simulink model "Modelo_R2023b"  (R2023b)
settings: Solver=VariableStepAuto  StartTime=0.0  StopTime=10.0  RelTol=1e-3
model workspace (MAT data in the model file):
  DC_Joint_J = 0.192319441127
  DC_Motor_D = 0.4
  DC_Motor_H = 0.192915716702
  DC_Motor_I = 1
  DC_Motor_J = 0.2131632295
  DC_Motor_Lower_Sat_Ref = -18
  DC_Motor_NLC = 0.11
  DC_Motor_NLS = 10000
  DC_Motor_P = 0.20625
  DC_Motor_ST = 0.0494309
  DC_Motor_TG = 0.95
  DC_Motor_Upper_Sat_Ref = 18
  DC_Motor_V = 12
  DRV_Deadzone_U = 128
  DRV_Motor_BTH = 0.001
  DRV_Motor_ETH = 0.15625
  DRV_Motor_FDR = 0.195188957589
  DRV_Motor_RTH = 0.001
  DRV_Motor_TBR = 0.10371374274
  MOTOR_Period_T = 0.01
  MOTOR_WHEEL_LPF : object (value not decoded)
  Robot_L = 0.15
  Robot_W = 0.15
  Robot_init_th = 0
  Robot_init_x = 0
  Robot_init_y = 0
  Robot_mm_to_m = 0.001
  Robot_wheel_radius = 0.05
  Robot_wheel_x_offset = 150
  Robot_wheel_y_offset = 102.5
  Robot_wheel_z_offset = 2
  Roller_Contact_df = 0.3
  Roller_Contact_dm = 1000
  Roller_Contact_sf = 0.5
  Roller_Contact_st = 1000000
  Roller_Joint_Friction = 0
  SIM_Base_Period_T = 0.001
  SIM_CTRL_Period_T = 0.1
  SIM_Floor_Height = 8.7
  SIM_Floor_Thick = 0.2
  SIM_Floor_Width = 9
  Sig : Simulink.Signal (value not decoded)
  Traj_ref = [0 0.1 0.2 0.3 0.4 0.5 0.6 0.7 0.8 0.9 1 0 ... (22 elements, 11x2)]
undefined symbols (not defined in the file): DiscIntNeverNeededParam, X, Y, Z
libraries: sm_lib x185, nesl_utility x37, fl_lib x32, ee_lib x12, simulink x8, aerolibconvert2 x4, cstblocks x4, sharedtransform x1, dspsigops x1
(part 2 of 4)

== system Modelo_R2023b/Nexus/World Frame with gravity ==
  Mechanism Configuration : sm_lib/Utilities/Mechanism Configuration  UniformGravity=Constant  GravityVector=[0 0 -9.80665]  GravityVectorUnits=m/s^2  LinearizationDelta=0.001  JointModeTransitionNonlinearIterations=2
  Solver Configuration : nesl_utility/Solver Configuration  PhysicalDomain=network_engine_domain  SubClassName=solver  LeftPortType=input  RightPortType=generic  Tones=[]  Harmonics=[]  SimulateNoise=off  Profile=off  UseLocalSampling=off  EnableSwitchedLinearOptims=on  FrequencyDomain=off  UseCCode=off  RelTol=0.001  AbsTol=1e-06  MinStep=1e-09  ToWorkspace=off  RevertToSquareIcSolve=off  NumHomotopyIterations=100  PhasorMode=off  PhasorModeNumHarmonics=1  ConsistencySolver=NEWTON_FTOL  IndexReductionMethod=DerivativeReplacement  DoDC=on  ResidualTolerance=1e-09  ConsistencyTolSource=GLOBAL  ConsistencyAbsTol=0.001  ConsistencyRelTol=0.001  ConsistencyTolFactor=0.001  UseLocalSolver=on  LocalSolverChoice=NE_PARTITIONING_ADVANCER  ResolveIndetEquations=on  FunctionEvalNumThread=1  LocalSolverSampleTime=0.001  DoFixedCost=off  MaxNonlinIter=3  MaxModeIter=2  ComputeImpulses=off  ImpulseIterations=2  LinearAlgebra=auto  LinearAlgebraNumThread=0  EquationFormulation=NE_TIME_EF  DelaysMemoryBudget=1024  AutomaticFiltering=off  FilteringTimeConstant=0.001  PartitionStorageMethod=AS_NEEDED  PartitionMemoryBudget=1024  PartitionMethod=FAST  MultibodyUseLocalSolver=off  MultibodyLocalSolverChoice=ODE1  MultibodyLocalSolverSampleTime=0.001
  World Frame : sm_lib/Frames and Transforms/World Frame
  WF : PMIOPort  Side=Right
  connections:
  Mechanism Configuration/RConn1 -- WF/RConn1 -- World Frame/RConn1 -- Solver Configuration/RConn1

== system Modelo_R2023b/Nexus/Nexus Robot/Sensors ==
  Frontal_Sonar_Sensor : sm_lib/Body Elements/File Solid  ExtGeomFileName=c_Nexus_Sonar_Sensor.stl  UnitType=Custom  ExtGeomFileUnits=mm  StepReaderType=HEX  ExportConvexHullGeometry=off  InertiaType=Custom  Mass=0  MassUnits=kg  CenterOfMass=[0, 0, 0]  CenterOfMassUnits=m  MomentsOfInertia=[0, 0, 0]  MomentsOfInertiaUnits=kg*m^2  ProductsOfInertia=[0, 0, 0]  ProductsOfInertiaUnits=kg*m^2  BasedOnType=DensityFromFile  Density=1000  DensityUnits=kg/m^3  DoExposeReferenceFrame=on  SerializedFrames=<Frames/>  GraphicType=FromGeometry  MarkerShape=Sphere  MarkerSize=10  GraphicVisPropType=SimpleVisualProperties  GraphicDiffuseColor=[0.15, 0.15, 0.15]  GraphicSpecularColor=[0.5 0.5 0.5 1.0]  GraphicAmbientColor=[0.15 0.15 0.15 1.0]  GraphicEmissiveColor=[0.0 0.0 0.0 1.0]  GraphicShininess=75  GraphicOpacity=1
  Left_Sonar_Sensor : sm_lib/Body Elements/File Solid  ExtGeomFileName=c_Nexus_Sonar_Sensor.stl  UnitType=Custom  ExtGeomFileUnits=mm  StepReaderType=HEX  ExportConvexHullGeometry=off  InertiaType=Custom  Mass=0  MassUnits=kg  CenterOfMass=[0, 0, 0]  CenterOfMassUnits=m  MomentsOfInertia=[0, 0, 0]  MomentsOfInertiaUnits=kg*m^2  ProductsOfInertia=[0, 0, 0]  ProductsOfInertiaUnits=kg*m^2  BasedOnType=DensityFromFile  Density=1000  DensityUnits=kg/m^3  DoExposeReferenceFrame=on  SerializedFrames=<Frames/>  GraphicType=FromGeometry  MarkerShape=Sphere  MarkerSize=10  GraphicVisPropType=SimpleVisualProperties  GraphicDiffuseColor=[0.15, 0.15, 0.15]  GraphicSpecularColor=[0.5 0.5 0.5 1.0]  GraphicAmbientColor=[0.15 0.15 0.15 1.0]  GraphicEmissiveColor=[0.0 0.0 0.0 1.0]  GraphicShininess=75  GraphicOpacity=1
  RT_Sensor_derecho : sm_lib/Frames and Transforms/Rigid Transform  TranslationMethod=Cartesian  TranslationStandardOffset=0  TranslationStandardOffsetUnits=m  TranslationStandardAxis=+Z  TranslationCartesianOffset=[0, -0.108, 0.01]  TranslationCartesianOffsetUnits=m  TranslationROffset=0  TranslationROffsetUnits=m  TranslationZOffset=0  TranslationZOffsetUnits=m  TranslationThetaOffset=0  TranslationThetaOffsetUnits=deg  RotationMethod=RotationSequence  RotationAngleUnits=deg  RotationStandardAxis=+Z  RotationAngle=0.0  RotationArbitraryAxis=[0 0 1]  FollAlignAxisA=+X  BaseAlignAxisA=+Y  FollAlignAxisB=+Y  BaseAlignAxisB=+Z  RotationSequenceAxes=BaseAxes  RotationSequence=ZYX  RotationSequenceAngles=[-90, 90, 0]  RotationSequenceAnglesUnits=deg  RotationMatrix=[1 0 0; 0 1 0; 0 0 1]  Quaternion=[1 0 0 0]
  RT_Sensor_frontal : sm_lib/Frames and Transforms/Rigid Transform  TranslationMethod=Cartesian  TranslationStandardOffset=0  TranslationStandardOffsetUnits=m  TranslationStandardAxis=+Z  TranslationCartesianOffset=[0.205, 0, 0.01]  TranslationCartesianOffsetUnits=m  TranslationROffset=0  TranslationROffsetUnits=m  TranslationZOffset=0  TranslationZOffsetUnits=m  TranslationThetaOffset=0  TranslationThetaOffsetUnits=deg  RotationMethod=RotationSequence  RotationAngleUnits=deg  RotationStandardAxis=+X  RotationAngle=90  RotationArbitraryAxis=[0 0 1]  FollAlignAxisA=+X  BaseAlignAxisA=+Y  FollAlignAxisB=+Y  BaseAlignAxisB=+Z  RotationSequenceAxes=BaseAxes  RotationSequence=ZYX  RotationSequenceAngles=[0, 0, 90]  RotationSequenceAnglesUnits=deg  RotationMatrix=[1 0 0; 0 1 0; 0 0 1]  Quaternion=[1 0 0 0]
  RT_Sensor_izquierdo : sm_lib/Frames and Transforms/Rigid Transform  TranslationMethod=Cartesian  TranslationStandardOffset=0  TranslationStandardOffsetUnits=m  TranslationStandardAxis=+Z  TranslationCartesianOffset=[0, 0.108, 0.01]  TranslationCartesianOffsetUnits=m  TranslationROffset=0  TranslationROffsetUnits=m  TranslationZOffset=0  TranslationZOffsetUnits=m  TranslationThetaOffset=0  TranslationThetaOffsetUnits=deg  RotationMethod=RotationSequence  RotationAngleUnits=deg  RotationStandardAxis=+X  RotationAngle=90  RotationArbitraryAxis=[0 0 1]  FollAlignAxisA=+Z  BaseAlignAxisA=+X  FollAlignAxisB=+Y  BaseAlignAxisB=+Y  RotationSequenceAxes=BaseAxes  RotationSequence=ZYX  RotationSequenceAngles=[90, 90, 0]  RotationSequenceAnglesUnits=deg  RotationMatrix=[1 0 0; 0 1 0; 0 0 1]  Quaternion=[1 0 0 0]
  RT_Sensor_trasero : sm_lib/Frames and Transforms/Rigid Transform  TranslationMethod=Cartesian  TranslationStandardOffset=0  TranslationStandardOffsetUnits=m  TranslationStandardAxis=+Z  TranslationCartesianOffset=[-0.201, 0, 0.01]  TranslationCartesianOffsetUnits=m  TranslationROffset=0  TranslationROffsetUnits=m  TranslationZOffset=0  TranslationZOffsetUnits=m  TranslationThetaOffset=0  TranslationThetaOffsetUnits=deg  RotationMethod=RotationSequence  RotationAngleUnits=deg  RotationStandardAxis=+Z  RotationAngle=0.0  RotationArbitraryAxis=[0 0 1]  FollAlignAxisA=+X  BaseAlignAxisA=+Y  FollAlignAxisB=+Y  BaseAlignAxisB=+Z  RotationSequenceAxes=BaseAxes  RotationSequence=ZYX  RotationSequenceAngles=[180, 0, 90]  RotationSequenceAnglesUnits=deg  RotationMatrix=[1 0 0; 0 1 0; 0 0 1]  Quaternion=[1 0 0 0]
  Rear_Sonar_Sensor : sm_lib/Body Elements/File Solid  ExtGeomFileName=c_Nexus_Sonar_Sensor.stl  UnitType=Custom  ExtGeomFileUnits=mm  StepReaderType=HEX  ExportConvexHullGeometry=off  InertiaType=Custom  Mass=0  MassUnits=kg  CenterOfMass=[0, 0, 0]  CenterOfMassUnits=m  MomentsOfInertia=[0, 0, 0]  MomentsOfInertiaUnits=kg*m^2  ProductsOfInertia=[0, 0, 0]  ProductsOfInertiaUnits=kg*m^2  BasedOnType=DensityFromFile  Density=1000  DensityUnits=kg/m^3  DoExposeReferenceFrame=on  SerializedFrames=<Frames/>  GraphicType=FromGeometry  MarkerShape=Sphere  MarkerSize=10  GraphicVisPropType=SimpleVisualProperties  GraphicDiffuseColor=[0.15, 0.15, 0.15]  GraphicSpecularColor=[0.5 0.5 0.5 1.0]  GraphicAmbientColor=[0.15 0.15 0.15 1.0]  GraphicEmissiveColor=[0.0 0.0 0.0 1.0]  GraphicShininess=75  GraphicOpacity=1
  Right_Sonar_Sensor : sm_lib/Body Elements/File Solid  ExtGeomFileName=c_Nexus_Sonar_Sensor.stl  UnitType=Custom  ExtGeomFileUnits=mm  StepReaderType=HEX  ExportConvexHullGeometry=off  InertiaType=Custom  Mass=0  MassUnits=kg  CenterOfMass=[0, 0, 0]  CenterOfMassUnits=m  MomentsOfInertia=[0, 0, 0]  MomentsOfInertiaUnits=kg*m^2  ProductsOfInertia=[0, 0, 0]  ProductsOfInertiaUnits=kg*m^2  BasedOnType=DensityFromFile  Density=1000  DensityUnits=kg/m^3  DoExposeReferenceFrame=on  SerializedFrames=<Frames/>  GraphicType=FromGeometry  MarkerShape=Sphere  MarkerSize=10  GraphicVisPropType=SimpleVisualProperties  GraphicDiffuseColor=[0.15, 0.15, 0.15]  GraphicSpecularColor=[0.5 0.5 0.5 1.0]  GraphicAmbientColor=[0.15 0.15 0.15 1.0]  GraphicEmissiveColor=[0.0 0.0 0.0 1.0]  GraphicShininess=75  GraphicOpacity=1
  F : PMIOPort  Side=Left
  connections:
  F/RConn1 -- RT_Sensor_derecho/LConn1 -- RT_Sensor_trasero/LConn1 -- RT_Sensor_izquierdo/LConn1 -- RT_Sensor_frontal/LConn1
  Frontal_Sonar_Sensor/RConn1 -- RT_Sensor_frontal/RConn1
  Left_Sonar_Sensor/RConn1 -- RT_Sensor_izquierdo/RConn1
  RT_Sensor_trasero/RConn1 -- Rear_Sonar_Sensor/RConn1
  RT_Sensor_derecho/RConn1 -- Right_Sonar_Sensor/RConn1

== system Modelo_R2023b/Nexus/Nexus Robot/Wheel ω1 Front Left ==
  ω1_ref : Inport
  DC_Motor Pololu 37DX70L 70:1 - 64 CPR : Subsystem
      settings: PortSchema="{\"entries\":[{\"content\":{\"sides\":[{\"content\":{\"connectorIds\":[\"In1\",\"LConn1\"]},\"type\":\"ConnectorPlacement.EquallySpacedRectSide\",\"uuid\":\"9ae33c20-e7ba-4d2e-ab0a-475af1e37d54\"},{\"content\":{\"connectorIds\":[\"RConn1\",\"Out1\"],\"side\":\"RIGHT\"},\"type\":\"ConnectorPlacement.EquallySpacedRectSide\",\"uuid\":\"3016d8d7-555e-445d-86be-78451b996395\"},{\"content\":{\"connectorIds\":[],\"side\":\"TOP\"},\"type\":\"ConnectorPlacement.EquallySpacedRectSide\",\"uuid\":\"fe670a4b-9c7a-4db9-8dc5-4a2b1004acda\"},{\"content\":{\"connectorIds\":[],\"side\":\"HIDDEN\"},\"type\":\"ConnectorPlacement.EquallySpacedRectSide\",\"uuid\":\"62c8cb45-536e-46ba-a998-0c96f5a31cbf\"}]},\"type\":\"ConnectorPlacement.EquallySpacedConnector\",\"uuid\":\"a5b4ceeb-7b8a-4016-b15f-272e7bc6952c\"}],\"packageUris\":[\"http://schema.mathworks.com/mf0/Connector/R2020b\"],\"version\":\"1.0\"}"
  Encoder : Subsystem  mask{CPR=4480*10, T_encoder=MOTOR_Period_T}
      mask prompts: CPR "Pulsos por vuelta"; T_encoder "Periodo de muestreo"
  LTI System1 : cstblocks/LTI System  sys=MOTOR_WHEEL_LPF  IC=[]  PadeOrder=0
  PID Controller : Subsystem
  Rate Transition : RateTransition
  Scope : Scope  NumInputPorts=3
  Wheel : Subsystem
  Zero-Order Hold1 : ZeroOrderHold  SampleTime=MOTOR_Period_T
  Zero-Order Hold4 : ZeroOrderHold  SampleTime=MOTOR_Period_T
  WC : PMIOPort  Side=Right
  FW : PMIOPort  Port=2  Side=Left
  ω1 : Outport
  wires:
  LTI System1/1 -> Scope/3, PID Controller/2(ω), ω1/1
  Zero-Order Hold4/1 -> Rate Transition/1
  Zero-Order Hold1/1 -> Encoder/1(In)
  Rate Transition/1 -> DC_Motor Pololu 37DX70L 70:1 - 64 CPR/1(U)
  ω1_ref/1 -> Scope/1, PID Controller/1(ω_ref)
  PID Controller/1(ω_u) -> Zero-Order Hold4/1
  DC_Motor Pololu 37DX70L 70:1 - 64 CPR/1(θ) -> Zero-Order Hold1/1
  Encoder/1(Out) -> LTI System1/1
  connections:
  WC/RConn1 -- Wheel/RConn1
  Wheel/LConn1 -- DC_Motor Pololu 37DX70L 70:1 - 64 CPR/RConn1
  FW/RConn1 -- DC_Motor Pololu 37DX70L 70:1 - 64 CPR/LConn1

== system Modelo_R2023b/Nexus/Nexus Robot/Wheel ω2 Front Right ==
  ω2_ref : Inport
  DC_Motor Pololu 37DX70L 70:1 - 64 CPR : Subsystem
      settings: PortSchema="{\"entries\":[{\"content\":{\"sides\":[{\"content\":{\"connectorIds\":[\"In1\",\"LConn1\"]},\"type\":\"ConnectorPlacement.EquallySpacedRectSide\",\"uuid\":\"9ae33c20-e7ba-4d2e-ab0a-475af1e37d54\"},{\"content\":{\"connectorIds\":[\"RConn1\",\"Out1\"],\"side\":\"RIGHT\"},\"type\":\"ConnectorPlacement.EquallySpacedRectSide\",\"uuid\":\"3016d8d7-555e-445d-86be-78451b996395\"},{\"content\":{\"connectorIds\":[],\"side\":\"TOP\"},\"type\":\"ConnectorPlacement.EquallySpacedRectSide\",\"uuid\":\"fe670a4b-9c7a-4db9-8dc5-4a2b1004acda\"},{\"content\":{\"connectorIds\":[],\"side\":\"HIDDEN\"},\"type\":\"ConnectorPlacement.EquallySpacedRectSide\",\"uuid\":\"62c8cb45-536e-46ba-a998-0c96f5a31cbf\"}]},\"type\":\"ConnectorPlacement.EquallySpacedConnector\",\"uuid\":\"a5b4ceeb-7b8a-4016-b15f-272e7bc6952c\"}],\"packageUris\":[\"http://schema.mathworks.com/mf0/Connector/R2020b\"],\"version\":\"1.0\"}"
  Encoder : Subsystem  mask{CPR=4480*10, T_encoder=MOTOR_Period_T}
      mask prompts: CPR "Pulsos por vuelta"; T_encoder "Periodo de muestreo"
  Gain1 : Gain  Gain=-1
  Gain2 : Gain  Gain=-1
  LTI System2 : cstblocks/LTI System  sys=MOTOR_WHEEL_LPF  IC=[]  PadeOrder=0
  PID Controller : Subsystem
  Rate Transition : RateTransition
  Wheel : Subsystem
  Zero-Order Hold1 : ZeroOrderHold  SampleTime=MOTOR_Period_T
  Zero-Order Hold3 : ZeroOrderHold  SampleTime=MOTOR_Period_T
  FW : PMIOPort  Side=Left
  WC : PMIOPort  Port=2  Side=Right
  ω2 : Outport
  wires:
  Rate Transition/1 -> DC_Motor Pololu 37DX70L 70:1 - 64 CPR/1(U)
  ω2_ref/1 -> Gain2/1
  Zero-Order Hold1/1 -> Encoder/1(In)
  Zero-Order Hold3/1 -> Rate Transition/1
  DC_Motor Pololu 37DX70L 70:1 - 64 CPR/1(θ) -> Zero-Order Hold1/1
  PID Controller/1(ω_u) -> Zero-Order Hold3/1
  Gain2/1 -> PID Controller/1(ω_ref)
  Encoder/1(Out) -> LTI System2/1
  Gain1/1 -> ω2/1
  LTI System2/1 -> PID Controller/2(ω), Gain1/1
  connections:
  Wheel/LConn1 -- DC_Motor Pololu 37DX70L 70:1 - 64 CPR/RConn1
  WC/RConn1 -- Wheel/RConn1
  FW/RConn1 -- DC_Motor Pololu 37DX70L 70:1 - 64 CPR/LConn1

== system Modelo_R2023b/Nexus/Nexus Robot/Wheel ω3 Back Left ==
  ω3_ref : Inport
  DC_Motor Pololu 37DX70L 70:1 - 64 CPR : Subsystem
      settings: PortSchema="{\"entries\":[{\"content\":{\"sides\":[{\"content\":{\"connectorIds\":[\"In1\",\"LConn1\"]},\"type\":\"ConnectorPlacement.EquallySpacedRectSide\",\"uuid\":\"9ae33c20-e7ba-4d2e-ab0a-475af1e37d54\"},{\"content\":{\"connectorIds\":[\"RConn1\",\"Out1\"],\"side\":\"RIGHT\"},\"type\":\"ConnectorPlacement.EquallySpacedRectSide\",\"uuid\":\"3016d8d7-555e-445d-86be-78451b996395\"},{\"content\":{\"connectorIds\":[],\"side\":\"TOP\"},\"type\":\"ConnectorPlacement.EquallySpacedRectSide\",\"uuid\":\"fe670a4b-9c7a-4db9-8dc5-4a2b1004acda\"},{\"content\":{\"connectorIds\":[],\"side\":\"HIDDEN\"},\"type\":\"ConnectorPlacement.EquallySpacedRectSide\",\"uuid\":\"62c8cb45-536e-46ba-a998-0c96f5a31cbf\"}]},\"type\":\"ConnectorPlacement.EquallySpacedConnector\",\"uuid\":\"a5b4ceeb-7b8a-4016-b15f-272e7bc6952c\"}],\"packageUris\":[\"http://schema.mathworks.com/mf0/Connector/R2020b\"],\"version\":\"1.0\"}"
  Encoder : Subsystem  mask{CPR=4480*10, T_encoder=MOTOR_Period_T}
      mask prompts: CPR "Pulsos por vuelta"; T_encoder "Periodo de muestreo"
  LTI System1 : cstblocks/LTI System  sys=MOTOR_WHEEL_LPF  IC=[]  PadeOrder=0
  PID Controller : Subsystem
  Rate Transition : RateTransition
  Wheel : Subsystem
  Zero-Order Hold1 : ZeroOrderHold  SampleTime=MOTOR_Period_T
  Zero-Order Hold3 : ZeroOrderHold  SampleTime=MOTOR_Period_T
  FW : PMIOPort  Side=Left
  WC : PMIOPort  Port=2  Side=Right
  ω3 : Outport
  wires:
  Rate Transition/1 -> DC_Motor Pololu 37DX70L 70:1 - 64 CPR/1(U)
  Zero-Order Hold1/1 -> Encoder/1(In)
  Zero-Order Hold3/1 -> Rate Transition/1
  DC_Motor Pololu 37DX70L 70:1 - 64 CPR/1(θ) -> Zero-Order Hold1/1
  PID Controller/1(ω_u) -> Zero-Order Hold3/1
  ω3_ref/1 -> PID Controller/1(ω_ref)
  Encoder/1(Out) -> LTI System1/1
  LTI System1/1 -> PID Controller/2(ω), ω3/1
  connections:
  Wheel/LConn1 -- DC_Motor Pololu 37DX70L 70:1 - 64 CPR/RConn1
  Wheel/RConn1 -- WC/RConn1
  FW/RConn1 -- DC_Motor Pololu 37DX70L 70:1 - 64 CPR/LConn1

== system Modelo_R2023b/Nexus/Nexus Robot/Wheel ω4 Back Right ==
  ω4_ref : Inport
  DC_Motor Pololu 37DX70L 70:1 - 64 CPR : Subsystem
      settings: PortSchema="{\"entries\":[{\"content\":{\"sides\":[{\"content\":{\"connectorIds\":[\"In1\",\"LConn1\"]},\"type\":\"ConnectorPlacement.EquallySpacedRectSide\",\"uuid\":\"9ae33c20-e7ba-4d2e-ab0a-475af1e37d54\"},{\"content\":{\"connectorIds\":[\"RConn1\",\"Out1\"],\"side\":\"RIGHT\"},\"type\":\"ConnectorPlacement.EquallySpacedRectSide\",\"uuid\":\"3016d8d7-555e-445d-86be-78451b996395\"},{\"content\":{\"connectorIds\":[],\"side\":\"TOP\"},\"type\":\"ConnectorPlacement.EquallySpacedRectSide\",\"uuid\":\"fe670a4b-9c7a-4db9-8dc5-4a2b1004acda\"},{\"content\":{\"connectorIds\":[],\"side\":\"HIDDEN\"},\"type\":\"ConnectorPlacement.EquallySpacedRectSide\",\"uuid\":\"62c8cb45-536e-46ba-a998-0c96f5a31cbf\"}]},\"type\":\"ConnectorPlacement.EquallySpacedConnector\",\"uuid\":\"a5b4ceeb-7b8a-4016-b15f-272e7bc6952c\"}],\"packageUris\":[\"http://schema.mathworks.com/mf0/Connector/R2020b\"],\"version\":\"1.0\"}"
  Encoder : Subsystem  mask{CPR=4480*10, T_encoder=MOTOR_Period_T}
      mask prompts: CPR "Pulsos por vuelta"; T_encoder "Periodo de muestreo"
  Gain1 : Gain  Gain=-1
  Gain2 : Gain  Gain=-1
  LTI System2 : cstblocks/LTI System  sys=MOTOR_WHEEL_LPF  IC=[]  PadeOrder=0
  PID Controller : Subsystem
  Rate Transition : RateTransition
  Wheel : Subsystem
  Zero-Order Hold1 : ZeroOrderHold  SampleTime=MOTOR_Period_T
  Zero-Order Hold3 : ZeroOrderHold  SampleTime=MOTOR_Period_T
  FW : PMIOPort  Side=Left
  WC : PMIOPort  Port=2  Side=Right
  ω4 : Outport
  wires:
  Rate Transition/1 -> DC_Motor Pololu 37DX70L 70:1 - 64 CPR/1(U)
  Zero-Order Hold1/1 -> Encoder/1(In)
  Zero-Order Hold3/1 -> Rate Transition/1
  DC_Motor Pololu 37DX70L 70:1 - 64 CPR/1(θ) -> Zero-Order Hold1/1
  PID Controller/1(ω_u) -> Zero-Order Hold3/1
  ω4_ref/1 -> Gain2/1
  LTI System2/1 -> PID Controller/2(ω), Gain1/1
  Gain2/1 -> PID Controller/1(ω_ref)
  Gain1/1 -> ω4/1
  Encoder/1(Out) -> LTI System2/1
  connections:
  Wheel/LConn1 -- DC_Motor Pololu 37DX70L 70:1 - 64 CPR/RConn1
  Wheel/RConn1 -- WC/RConn1
  FW/RConn1 -- DC_Motor Pololu 37DX70L 70:1 - 64 CPR/LConn1

== system Modelo_R2023b/Nexus/Walls/Beacon_1 ==
  Beacon_1 : sm_lib/Body Elements/File Solid  ExtGeomFileName=c_Beacon.stl  UnitType=Custom  ExtGeomFileUnits=mm  StepReaderType=HEX  ExportConvexHullGeometry=off  InertiaType=PointMass  Mass=59  MassUnits=g  CenterOfMass=[0 0 0]  CenterOfMassUnits=m  MomentsOfInertia=[1 1 1]  MomentsOfInertiaUnits=kg*m^2  ProductsOfInertia=[0 0 0]  ProductsOfInertiaUnits=kg*m^2  BasedOnType=Mass  Density=1000  DensityUnits=kg/m^3  DoExposeReferenceFrame=on  SerializedFrames=<Frames/>  GraphicType=FromGeometry  MarkerShape=Sphere  MarkerSize=10  GraphicVisPropType=SimpleVisualProperties  GraphicDiffuseColor=[0.0 1.0 1.0]  GraphicSpecularColor=[0.5 0.5 0.5 1.0]  GraphicAmbientColor=[0.15 0.15 0.15 1.0]  GraphicEmissiveColor=[0.0 0.0 0.0 1.0]  GraphicShininess=75  GraphicOpacity=1.0
  Rigid Transform1 : sm_lib/Frames and Transforms/Rigid Transform  TranslationMethod=Cartesian  TranslationStandardOffset=0  TranslationStandardOffsetUnits=cm  TranslationStandardAxis=+Z  TranslationCartesianOffset=[(-20+24.5+3) 5 -5]  TranslationCartesianOffsetUnits=cm  TranslationROffset=0  TranslationROffsetUnits=m  TranslationZOffset=0  TranslationZOffsetUnits=m  TranslationThetaOffset=0  TranslationThetaOffsetUnits=deg  RotationMethod=StandardAxis  RotationAngleUnits=deg  RotationStandardAxis=-Y  RotationAngle=90  RotationArbitraryAxis=[0 0 1]  FollAlignAxisA=+X  BaseAlignAxisA=+Y  FollAlignAxisB=+Y  BaseAlignAxisB=+Z  RotationSequenceAxes=FollowerAxes  RotationSequence=XYX  RotationSequenceAngles=[0 0 0]  RotationSequenceAnglesUnits=deg  RotationMatrix=[1 0 0; 0 1 0; 0 0 1]  Quaternion=[1 0 0 0]
  FT : PMIOPort  Side=Left
  F : PMIOPort  Port=2  Side=Right
  connections:
  Rigid Transform1/RConn1 -- F/RConn1
  Rigid Transform1/LConn1 -- FT/RConn1 -- Beacon_1/RConn1

== system Modelo_R2023b/Nexus/Walls/Beacon_2 ==
  Beacon_2 : sm_lib/Body Elements/File Solid  ExtGeomFileName=c_Beacon.stl  UnitType=Custom  ExtGeomFileUnits=mm  StepReaderType=HEX  ExportConvexHullGeometry=off  InertiaType=PointMass  Mass=59  MassUnits=g  CenterOfMass=[0 0 0]  CenterOfMassUnits=m  MomentsOfInertia=[1 1 1]  MomentsOfInertiaUnits=kg*m^2  ProductsOfInertia=[0 0 0]  ProductsOfInertiaUnits=kg*m^2  BasedOnType=Mass  Density=1000  DensityUnits=kg/m^3  DoExposeReferenceFrame=on  SerializedFrames=<Frames/>  GraphicType=FromGeometry  MarkerShape=Sphere  MarkerSize=10  GraphicVisPropType=SimpleVisualProperties  GraphicDiffuseColor=[0.0 1.0 1.0]  GraphicSpecularColor=[0.5 0.5 0.5 1.0]  GraphicAmbientColor=[0.15 0.15 0.15 1.0]  GraphicEmissiveColor=[0.0 0.0 0.0 1.0]  GraphicShininess=75  GraphicOpacity=1.0
  Rigid Transform1 : sm_lib/Frames and Transforms/Rigid Transform  TranslationMethod=Cartesian  TranslationStandardOffset=0  TranslationStandardOffsetUnits=cm  TranslationStandardAxis=+Z  TranslationCartesianOffset=[(20-24.5-3) 5 -5]  TranslationCartesianOffsetUnits=cm  TranslationROffset=0  TranslationROffsetUnits=m  TranslationZOffset=0  TranslationZOffsetUnits=m  TranslationThetaOffset=0  TranslationThetaOffsetUnits=deg  RotationMethod=StandardAxis  RotationAngleUnits=deg  RotationStandardAxis=+Y  RotationAngle=90  RotationArbitraryAxis=[0 0 1]  FollAlignAxisA=+X  BaseAlignAxisA=+Y  FollAlignAxisB=+Y  BaseAlignAxisB=+Z  RotationSequenceAxes=FollowerAxes  RotationSequence=XYX  RotationSequenceAngles=[0 0 0]  RotationSequenceAnglesUnits=deg  RotationMatrix=[1 0 0; 0 1 0; 0 0 1]  Quaternion=[1 0 0 0]
  FT : PMIOPort  Side=Left
  F : PMIOPort  Port=2  Side=Right
  connections:
  Rigid Transform1/RConn1 -- F/RConn1
  FT/RConn1 -- Rigid Transform1/LConn1 -- Beacon_2/RConn1

== system Modelo_R2023b/Nexus/Walls/Beacon_3 ==
  Beacon_3 : sm_lib/Body Elements/File Solid  ExtGeomFileName=c_Beacon.stl  UnitType=Custom  ExtGeomFileUnits=mm  StepReaderType=HEX  ExportConvexHullGeometry=off  InertiaType=PointMass  Mass=59  MassUnits=g  CenterOfMass=[0 0 0]  CenterOfMassUnits=m  MomentsOfInertia=[1 1 1]  MomentsOfInertiaUnits=kg*m^2  ProductsOfInertia=[0 0 0]  ProductsOfInertiaUnits=kg*m^2  BasedOnType=Mass  Density=1000  DensityUnits=kg/m^3  DoExposeReferenceFrame=on  SerializedFrames=<Frames/>  GraphicType=FromGeometry  MarkerShape=Sphere  MarkerSize=10  GraphicVisPropType=SimpleVisualProperties  GraphicDiffuseColor=[0.0 1.0 1.0]  GraphicSpecularColor=[0.5 0.5 0.5 1.0]  GraphicAmbientColor=[0.15 0.15 0.15 1.0]  GraphicEmissiveColor=[0.0 0.0 0.0 1.0]  GraphicShininess=75  GraphicOpacity=1.0
  Rigid Transform1 : sm_lib/Frames and Transforms/Rigid Transform  TranslationMethod=Cartesian  TranslationStandardOffset=0  TranslationStandardOffsetUnits=cm  TranslationStandardAxis=+Z  TranslationCartesianOffset=[0 (20-24.5-3) -5]  TranslationCartesianOffsetUnits=cm  TranslationROffset=0  TranslationROffsetUnits=m  TranslationZOffset=0  TranslationZOffsetUnits=m  TranslationThetaOffset=0  TranslationThetaOffsetUnits=deg  RotationMethod=StandardAxis  RotationAngleUnits=deg  RotationStandardAxis=-X  RotationAngle=90  RotationArbitraryAxis=[0 0 1]  FollAlignAxisA=+X  BaseAlignAxisA=+Y  FollAlignAxisB=+Y  BaseAlignAxisB=+Z  RotationSequenceAxes=FollowerAxes  RotationSequence=XYX  RotationSequenceAngles=[0 0 0]  RotationSequenceAnglesUnits=deg  RotationMatrix=[1 0 0; 0 1 0; 0 0 1]  Quaternion=[1 0 0 0]
  FT : PMIOPort  Side=Left
  F : PMIOPort  Port=2  Side=Right
  connections:
  Rigid Transform1/RConn1 -- F/RConn1
  FT/RConn1 -- Rigid Transform1/LConn1 -- Beacon_3/RConn1

== system Modelo_R2023b/Nexus/Walls/Beacon_4 ==
  Beacon_4 : sm_lib/Body Elements/File Solid  ExtGeomFileName=c_Beacon.stl  UnitType=Custom  ExtGeomFileUnits=mm  StepReaderType=HEX  ExportConvexHullGeometry=off  InertiaType=PointMass  Mass=59  MassUnits=g  CenterOfMass=[0 0 0]  CenterOfMassUnits=m  MomentsOfInertia=[1 1 1]  MomentsOfInertiaUnits=kg*m^2  ProductsOfInertia=[0 0 0]  ProductsOfInertiaUnits=kg*m^2  BasedOnType=Mass  Density=1000  DensityUnits=kg/m^3  DoExposeReferenceFrame=on  SerializedFrames=<Frames/>  GraphicType=FromGeometry  MarkerShape=Sphere  MarkerSize=10  GraphicVisPropType=SimpleVisualProperties  GraphicDiffuseColor=[0.0 1.0 1.0]  GraphicSpecularColor=[0.5 0.5 0.5 1.0]  GraphicAmbientColor=[0.15 0.15 0.15 1.0]  GraphicEmissiveColor=[0.0 0.0 0.0 1.0]  GraphicShininess=75  GraphicOpacity=1.0
  Rigid Transform1 : sm_lib/Frames and Transforms/Rigid Transform  TranslationMethod=Cartesian  TranslationStandardOffset=0  TranslationStandardOffsetUnits=cm  TranslationStandardAxis=+Z  TranslationCartesianOffset="[0  (-20+24.5+3) -5]"  TranslationCartesianOffsetUnits=cm  TranslationROffset=0  TranslationROffsetUnits=m  TranslationZOffset=0  TranslationZOffsetUnits=m  TranslationThetaOffset=0  TranslationThetaOffsetUnits=deg  RotationMethod=StandardAxis  RotationAngleUnits=deg  RotationStandardAxis=+X  RotationAngle=90  RotationArbitraryAxis=[0 0 1]  FollAlignAxisA=+X  BaseAlignAxisA=+Y  FollAlignAxisB=+Y  BaseAlignAxisB=+Z  RotationSequenceAxes=FollowerAxes  RotationSequence=XYX  RotationSequenceAngles=[0 0 0]  RotationSequenceAnglesUnits=deg  RotationMatrix=[1 0 0; 0 1 0; 0 0 1]  Quaternion=[1 0 0 0]
  FT : PMIOPort  Side=Left
  F : PMIOPort  Port=2  Side=Right
  connections:
  Rigid Transform1/RConn1 -- F/RConn1
  FT/RConn1 -- Rigid Transform1/LConn1 -- Beacon_4/RConn1

== system Modelo_R2023b/Nexus/Nexus Robot/Wheel ω1 Front Left/DC_Motor Pololu 37DX70L 70:1 - 64 CPR ==
  U : Inport
  Angle Conversion : aerolibconvert2/Angle Conversion  IU=deg  OU=rad
  Electrical : Subsystem  mask{nomV=12}
      mask prompts: nomV "Nominal Voltage (V)"
  Mechanics : Subsystem
  PS-Simulink Converter : nesl_utility/PS-Simulink Converter  PhysicalDomain=network_engine_domain  SubClassName=ps_output  LeftPortType=input  RightPortType=output  PseudoPeriodic=off  Frequencies=[]  VectorFormat=1-D array  Unit=deg  AffineConversion=off
  PS-Simulink Converter1 : nesl_utility/PS-Simulink Converter  PhysicalDomain=network_engine_domain  SubClassName=ps_output  LeftPortType=input  RightPortType=output  PseudoPeriodic=off  Frequencies=[]  VectorFormat=1-D array  Unit=rad/s  AffineConversion=off
  PS-Simulink Converter2 : nesl_utility/PS-Simulink Converter  PhysicalDomain=network_engine_domain  SubClassName=ps_output  LeftPortType=input  RightPortType=output  PseudoPeriodic=off  Frequencies=[]  VectorFormat=1-D array  Unit=N*m  AffineConversion=off
  PS-Simulink Converter3 : nesl_utility/PS-Simulink Converter  PhysicalDomain=network_engine_domain  SubClassName=ps_output  LeftPortType=input  RightPortType=output  PseudoPeriodic=off  Frequencies=[]  VectorFormat=1-D array  Unit=A  AffineConversion=off
  Terminator : Terminator
  Terminator1 : Terminator
  Terminator2 : Terminator
  FW : PMIOPort  Side=Left
  Wheel : PMIOPort  Port=2  Side=Right
  θ : Outport
  wires:
  PS-Simulink Converter/1 -> Angle Conversion/1
  Angle Conversion/1 -> θ/1
  U/1 -> Electrical/1(U)
  PS-Simulink Converter1/1 -> Terminator/1
  PS-Simulink Converter2/1 -> Terminator1/1
  PS-Simulink Converter3/1 -> Terminator2/1
  connections:
  PS-Simulink Converter3/LConn1 -- Electrical/RConn2
  PS-Simulink Converter/LConn1 -- Mechanics/RConn2
  PS-Simulink Converter1/LConn1 -- Mechanics/RConn3
  Electrical/RConn1 -- PS-Simulink Converter2/LConn1 -- Mechanics/LConn2
  Mechanics/LConn1 -- FW/RConn1
  Wheel/RConn1 -- Mechanics/RConn1

== system Modelo_R2023b/Nexus/Nexus Robot/Wheel ω1 Front Left/Encoder ==
  In : Inport
  Difference : simulink/Discrete/Difference  ICPrevInput=0.0  OutMin=[]  OutMax=[]  OutDataType=fixdt(1, 16)  OutScaling=2^-10  DoSatur=off
  Gain : Gain  Gain=CPR/(2*pi)
  Gain1 : Gain  Gain=(2*pi)/CPR
  Gain2 : Gain  Gain=1/T_encoder
  Round : Rounding  Operator=fix
  Out : Outport
  wires:
  Round/1 -> Gain1/1
  Gain/1 -> Round/1
  Gain1/1 -> Difference/1
  In/1 -> Gain/1
  Difference/1 -> Gain2/1
  Gain2/1 -> Out/1

== system Modelo_R2023b/Nexus/Nexus Robot/Wheel ω1 Front Left/PID Controller ==
  ω_ref : Inport
  ω : Inport  Port=2
  Discrete Derivative : simulink/Discrete/Discrete Derivative  gainval=1.0  ICPrevScaledInput=0.0  OutMin=[]  OutMax=[]  OutDataType=fixdt(1, 16)  OutScaling=2^-10  DoSatur=off
  Discrete-Time Integrator1 : DiscreteIntegrator  SampleTime=MOTOR_Period_T  ICPrevOutput=DiscIntNeverNeededParam  ICPrevScaledInput=DiscIntNeverNeededParam
  Gain : Gain  Gain=4096/12
  Gain1 : Gain  Gain=DC_Motor_P
  Gain2 : Gain  Gain=DC_Motor_I
  Gain3 : Gain  Gain=DC_Motor_D
  Sum : Sum  Inputs=+-|
  Sum1 : Sum  Inputs=+++
  ω_u : Outport
  wires:
  Gain/1 -> ω_u/1
  ω/1 -> Sum/2
  Gain2/1 -> Discrete-Time Integrator1/1
  Sum/1 -> Gain3/1, Gain1/1, Gain2/1  "error"
  Sum1/1 -> Gain/1  "ω_v"
  ω_ref/1 -> Sum/1
  Discrete-Time Integrator1/1 -> Sum1/2
  Gain1/1 -> Sum1/1
  Discrete Derivative/1 -> Sum1/3
  Gain3/1 -> Discrete Derivative/1

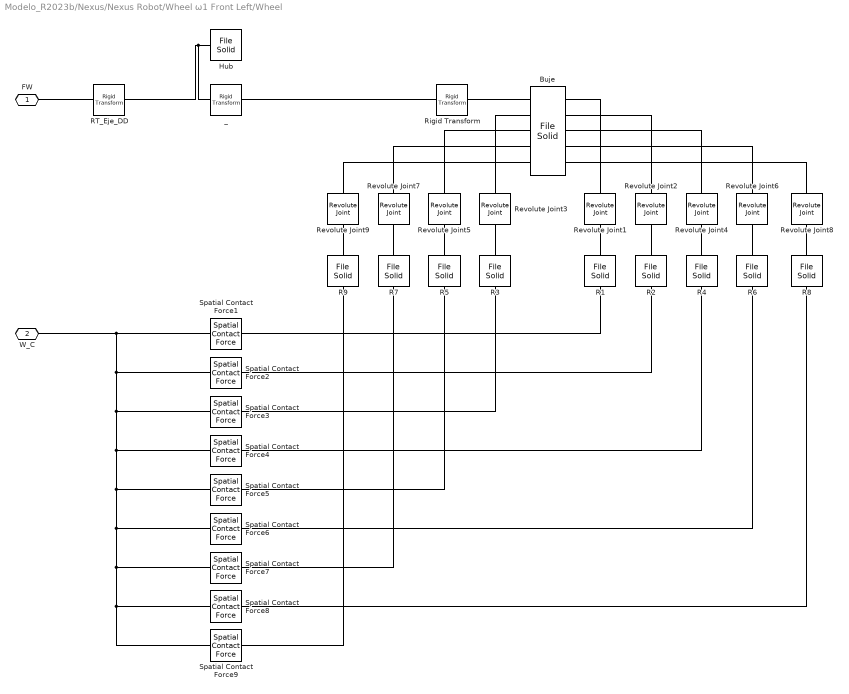
== system Modelo_R2023b/Nexus/Nexus Robot/Wheel ω1 Front Left/Wheel ==
  Buje : sm_lib/Body Elements/File Solid  ExtGeomFileName=c_Nexus_Wheel_B.stp  UnitType=FromFile  ExtGeomFileUnits=m  StepReaderType=HEX  ExportConvexHullGeometry=off  InertiaType=CalculateFromGeometry  Mass=200  MassUnits=g  CenterOfMass=[0 0 0]  CenterOfMassUnits=m  MomentsOfInertia=[1 1 1]  MomentsOfInertiaUnits=kg*m^2  ProductsOfInertia=[1 1 1]  ProductsOfInertiaUnits=kg*m^2  BasedOnType=Mass  Density=196  DensityUnits=g/cm^3  DoExposeReferenceFrame=on  SerializedFrames=<Frames><Frame><Id>Frame1</Id><Value><Name>F1</Name><Origin><Source>GeometricFeature</Source><FeatureName>circular curve 129</FeatureName></Origin><PrimaryAxis><DefinedDirection>+Z</DefinedDirection><Source>GeometricFeature</Source><SourceDirection>+Z</SourceDirection><FeatureName>circular curve 129</FeatureName></PrimaryAxis><SecondaryAxis><DefinedDirection>+X</DefinedDirection><Source>ReferenceFrame</Source><SourceDirection>+X</SourceDirection><FeatureName></FeatureName></SecondaryAxis></Value></Frame><Frame><Id>Frame2</Id><Value><Name>F2</Name><Origin><Source>GeometricFeature</Source><FeatureName>circular curve 133</FeatureName></Origin><PrimaryAxis><DefinedDirection>+Z</DefinedDirection><Source>GeometricFeature</Source><SourceDirection>+Z</SourceDirection><FeatureName>circular curve 133</FeatureName></PrimaryAxis><SecondaryAxis><DefinedDirection>+X</DefinedDirection><Source>ReferenceFrame</Source><SourceDirection>+X</SourceDirection><FeatureName></FeatureName></SecondaryAxis></Value></Frame><Frame><Id>Frame3</Id><Value><Name>F3</Name><Origin><Source>GeometricFeature</Source><FeatureName>circular curve 137</FeatureName></Origin><PrimaryAxis><DefinedDirection>+Z</DefinedDirection><Source>GeometricFeature</Source><SourceDirection>+Z</SourceDirection><FeatureName>circular curve 137</FeatureName></PrimaryAxis><SecondaryAxis><DefinedDirection>+X</DefinedDirection><Source>ReferenceFrame</Source><SourceDirection>+X</SourceDirection><FeatureName></FeatureName></SecondaryAxis></Value></Frame><Frame><Id>Frame4</Id><Value><Name>F4</Name><Origin><Source>GeometricFeature</Source><FeatureName>circular curve 141</FeatureName></Origin><PrimaryAxis><DefinedDirection>+Z</DefinedDirection><Source>GeometricFeature</Source><SourceDirection>+Z</SourceDirection><FeatureName>circular curve 141</FeatureName></PrimaryAxis><SecondaryAxis><DefinedDirection>+X</DefinedDirection><Source>ReferenceFrame</Source><SourceDirection>+X</SourceDirection><FeatureName></FeatureName></SecondaryAxis></Value></Frame><Frame><Id>Frame5</Id><Value><Name>F5</Name><Origin><Source>GeometricFeature</Source><FeatureName>circular curve 147</FeatureName></Origin><PrimaryAxis><DefinedDirection>+Z</DefinedDirection><Source>GeometricFeature</Source><SourceDirection>+Z</SourceDirection><FeatureName>circular curve 147</FeatureName></PrimaryAxis><SecondaryAxis><DefinedDirection>+X</DefinedDirection><Source>ReferenceFrame</Source><SourceDirection>+X</SourceDirection><FeatureName></FeatureName></SecondaryAxis></Value></Frame><Frame><Id>Frame6</Id><Value><Name>F6</Name><Origin><Source>GeometricFeature</Source><FeatureName>circular curve 153</FeatureName></Origin><PrimaryAxis><DefinedDirection>+Z</DefinedDirection><Source>GeometricFeature</Source><SourceDirection>+Z</SourceDirection><FeatureName>circular curve 153</FeatureName></PrimaryAxis><SecondaryAxis><DefinedDirection>+X</DefinedDirection><Source>ReferenceFrame</Source><SourceDirection>+X</SourceDirection><FeatureName></FeatureName></SecondaryAxis></Value></Frame><Frame><Id>Frame7</Id><Value><Name>F7</Name><Origin><Source>GeometricFeature</Source><FeatureName>circular curve 159</FeatureName></Origin><PrimaryAxis><DefinedDirection>+Z</DefinedDirection><Source>GeometricFeature</Source><SourceDirection>+Z</SourceDirection><FeatureName>circular curve 159</FeatureName></PrimaryAxis><SecondaryAxis><DefinedDirection>+X</DefinedDirection><Source>ReferenceFrame</Source><SourceDirection>+X</SourceDirection><FeatureName></FeatureName></SecondaryAxis></Value></Frame><Frame><Id>Frame8</Id><Value><Name>F8</Name><Origin><Source>GeometricFeature</Source><FeatureName>circular curve 165</FeatureName></Origin><PrimaryAxis><DefinedDirection>+Z</DefinedDirection><Source>GeometricFeature</Source><SourceDirection>+Z</SourceDirection><FeatureName>circular curve 165</FeatureName></PrimaryAxis><SecondaryAxis><DefinedDirection>+X</DefinedDirection><Source>ReferenceFrame</Source><SourceDirection>+X</SourceDirection><FeatureName></FeatureName></SecondaryAxis></Value></Frame><Frame><Id>Frame9</Id><Value><Name>F9</Name><Origin><Source>GeometricFeature</Source><FeatureName>circular curve 169</FeatureName></Origin><PrimaryAxis><DefinedDirection>+Z</DefinedDirection><Source>GeometricFeature</Source><SourceDirection>+Z</SourceDirection><FeatureName>circular curve 169</FeatureName></PrimaryAxis><SecondaryAxis><DefinedDirection>+X</DefinedDirection><Source>ReferenceFrame</Source><SourceDirection>+X</SourceDirection><FeatureName></FeatureName></SecondaryAxis></Value></Frame></Frames>  GraphicType=FromGeometry  MarkerShape=Sphere  MarkerSize=10  GraphicVisPropType=SimpleVisualProperties  GraphicDiffuseColor=[0.8 1.0 1.0]  GraphicSpecularColor=[0.5 0.5 0.5 1.0]  GraphicAmbientColor=[0.15 0.15 0.15 1.0]  GraphicEmissiveColor=[0.0 0.0 0.0 1.0]  GraphicShininess=75  GraphicOpacity=1.0
  Hub : sm_lib/Body Elements/File Solid  ExtGeomFileName=c_Nexus_Wheel_Shaft.stl  UnitType=Custom  ExtGeomFileUnits=mm  StepReaderType=HEX  ExportConvexHullGeometry=off  InertiaType=Custom  Mass=0  MassUnits=kg  CenterOfMass=[0, 0, 0]  CenterOfMassUnits=m  MomentsOfInertia=[0, 0, 0]  MomentsOfInertiaUnits=kg*m^2  ProductsOfInertia=[0, 0, 0]  ProductsOfInertiaUnits=kg*m^2  BasedOnType=DensityFromFile  Density=1000  DensityUnits=kg/m^3  DoExposeReferenceFrame=on  SerializedFrames=<Frames/>  GraphicType=FromGeometry  MarkerShape=Sphere  MarkerSize=10  GraphicVisPropType=SimpleVisualProperties  GraphicDiffuseColor=[0.0 0.0 0.0]  GraphicSpecularColor=[0.5 0.5 0.5 1.0]  GraphicAmbientColor=[0.15 0.15 0.15 1.0]  GraphicEmissiveColor=[0.0 0.0 0.0 1.0]  GraphicShininess=75  GraphicOpacity=1
  R{1..9} (9 alike) : sm_lib/Body Elements/File Solid  ExtGeomFileName=c_Nexus_Wheel_Roller.stp  UnitType=FromFile  ExtGeomFileUnits=m  StepReaderType=HEX  ExportConvexHullGeometry=on  InertiaType=CalculateFromGeometry  Mass=1  MassUnits=kg  CenterOfMass=[0 0 0]  CenterOfMassUnits=m  MomentsOfInertia=[1 1 1]  MomentsOfInertiaUnits=kg*m^2  ProductsOfInertia=[1 1 1]  ProductsOfInertiaUnits=kg*m^2  BasedOnType=Density  Density=1000  DensityUnits=kg/m^3  DoExposeReferenceFrame=on  SerializedFrames=<Frames/>  GraphicType=FromGeometry  MarkerShape=Sphere  MarkerSize=10  GraphicVisPropType=SimpleVisualProperties  GraphicDiffuseColor=[0.0 0.0 0.0]  GraphicSpecularColor=[0.5 0.5 0.5 1.0]  GraphicAmbientColor=[0.15 0.15 0.15 1.0]  GraphicEmissiveColor=[0.0 0.0 0.0 1.0]  GraphicShininess=75  GraphicOpacity=1.0
  RT_Eje_DD : sm_lib/Frames and Transforms/Rigid Transform  TranslationMethod=Cartesian  TranslationStandardOffset=0  TranslationStandardOffsetUnits=mm  TranslationStandardAxis=+Z  TranslationCartesianOffset=[0, 0, -10]  TranslationCartesianOffsetUnits=mm  TranslationROffset=0  TranslationROffsetUnits=m  TranslationZOffset=0  TranslationZOffsetUnits=m  TranslationThetaOffset=0  TranslationThetaOffsetUnits=deg  RotationMethod=RotationSequence  RotationAngleUnits=deg  RotationStandardAxis=+Z  RotationAngle=0.0  RotationArbitraryAxis=[0 0 1]  FollAlignAxisA=+X  BaseAlignAxisA=+Y  FollAlignAxisB=+Y  BaseAlignAxisB=+Z  RotationSequenceAxes=BaseAxes  RotationSequence=ZYX  RotationSequenceAngles=[90, 90, 0]  RotationSequenceAnglesUnits=deg  RotationMatrix=[1 0 0; 0 1 0; 0 0 1]  Quaternion=[1 0 0 0]
  Revolute Joint{1..9} (9 alike) : sm_lib/Joints/Revolute Joint  JointMode=Normal  SenseConstraintForce=off  SenseConstraintForceX=off  SenseConstraintForceY=off  SenseConstraintForceZ=off  SenseConstraintTorque=off  SenseConstraintTorqueX=off  SenseConstraintTorqueY=off  SenseConstraintTorqueZ=off  SenseTotalForce=off  SenseTotalForceX=off  SenseTotalForceY=off  SenseTotalForceZ=off  SenseTotalTorque=off  SenseTotalTorqueX=off  SenseTotalTorqueY=off  SenseTotalTorqueZ=off  CompositeWrenchDir=FollowerOnBase  CompositeWrenchFrame=BaseFrame  EquilibriumPosition=0  EquilibriumPositionUnits=deg  SpringStiffness=0  SpringStiffnessUnits=N*m/deg  DampingCoefficient=Roller_Joint_Friction  DampingCoefficientUnits=N*m/(deg/s)  TorqueActuationMode=NoTorque  MotionActuationMode=ComputedMotion  SensePosition=off  SenseVelocity=off  SenseAcceleration=off  SenseTorqueForce=off  SenseLowerLimitTorqueForce=off  SenseUpperLimitTorqueForce=off  LowerLimitSpecify=off  LowerLimitBound=-90  LowerLimitBoundUnits=deg  LowerLimitStiffness=1e4  LowerLimitStiffnessUnits=N*m/deg  LowerLimitDamping=10  LowerLimitDampingUnits=N*m/(deg/s)  LowerLimitTransitionRegionWidth=0.1  LowerLimitTransitionRegionWidthUnits=deg  UpperLimitSpecify=off  UpperLimitBound=90  UpperLimitBoundUnits=deg  UpperLimitStiffness=1e4  UpperLimitStiffnessUnits=N*m/deg  UpperLimitDamping=10  UpperLimitDampingUnits=N*m/(deg/s)  UpperLimitTransitionRegionWidth=0.1  UpperLimitTransitionRegionWidthUnits=deg  PositionTargetSpecify=off  PositionTargetPriority=High  PositionTargetValue=0  PositionTargetValueUnits=deg  VelocityTargetSpecify=off  VelocityTargetPriority=High  VelocityTargetValue=0  VelocityTargetValueUnits=deg/s
  Rigid Transform : sm_lib/Frames and Transforms/Rigid Transform  TranslationMethod=Cartesian  TranslationStandardOffset=0  TranslationStandardOffsetUnits=m  TranslationStandardAxis=+Z  TranslationCartesianOffset=[0 0 0.015]  TranslationCartesianOffsetUnits=m  TranslationROffset=0  TranslationROffsetUnits=m  TranslationZOffset=0  TranslationZOffsetUnits=m  TranslationThetaOffset=0  TranslationThetaOffsetUnits=deg  RotationMethod=StandardAxis  RotationAngleUnits=deg  RotationStandardAxis=+Y  RotationAngle=-90  RotationArbitraryAxis=[0 0 1]  FollAlignAxisA=+X  BaseAlignAxisA=+Y  FollAlignAxisB=+Y  BaseAlignAxisB=+Z  RotationSequenceAxes=FollowerAxes  RotationSequence=XYX  RotationSequenceAngles=[0 0 0]  RotationSequenceAnglesUnits=deg  RotationMatrix=[1 0 0; 0 1 0; 0 0 1]  Quaternion=[1 0 0 0]
  Spatial Contact Force{1..9} (9 alike) : sm_lib/Forces and Torques/Spatial Contact Force  SenseContactBaseRotation=off  SenseContactBaseTranslation=off  CoefficientOfDynamicFriction=Roller_Contact_df  CoefficientOfStaticFriction=Roller_Contact_sf  NormalDamping=Roller_Contact_dm  NormalDampingUnits=N/(m/s)  SenseContactSignal=off  NormalStiffness=Roller_Contact_st  NormalStiffnessUnits=N/m  FrictionalCriticalVelocity=1e-3  FrictionalCriticalVelocityUnits=m/s  ZeroCrossDetectContactStartAndEnd=off  SenseContactFollowerRotation=off  SenseContactFollowerTranslation=off  FrictionType=SmoothStickSlip  SenseFrictionalForceMagnitude=off  SenseNormalForceMagnitude=off  NormalForceType=SmoothSpringDamper  SenseNormalVelocity=off  SensePenetrationDepth=off  SenseSeparationDistance=off  SenseTangentialVelocity=off  NormalTransitionRegionWidth=1e-4  NormalTransitionRegionWidthUnits=m
  _ : sm_lib/Frames and Transforms/Rigid Transform  TranslationMethod=Cartesian  TranslationStandardOffset=0  TranslationStandardOffsetUnits=m  TranslationStandardAxis=+Z  TranslationCartesianOffset=[0, 0.042+0.009, 0]  TranslationCartesianOffsetUnits=m  TranslationROffset=0  TranslationROffsetUnits=m  TranslationZOffset=0  TranslationZOffsetUnits=m  TranslationThetaOffset=0  TranslationThetaOffsetUnits=deg  RotationMethod=StandardAxis  RotationAngleUnits=deg  RotationStandardAxis=+X  RotationAngle=-90  RotationArbitraryAxis=[0 0 1]  FollAlignAxisA=+X  BaseAlignAxisA=+Y  FollAlignAxisB=+Y  BaseAlignAxisB=+Z  RotationSequenceAxes=BaseAxes  RotationSequence=ZYX  RotationSequenceAngles=[180, 0, 0]  RotationSequenceAnglesUnits=deg  RotationMatrix=[1 0 0; 0 1 0; 0 0 1]  Quaternion=[1 0 0 0]
  FW : PMIOPort  Side=Left
  W_C : PMIOPort  Port=2  Side=Right
  connections:
  Hub/RConn1 -- RT_Eje_DD/RConn1 -- _/LConn1
  RT_Eje_DD/LConn1 -- FW/RConn1
  Spatial Contact Force1/LConn1 -- W_C/RConn1 -- Spatial Contact Force2/LConn1 -- Spatial Contact Force3/LConn1 -- Spatial Contact Force4/LConn1 -- Spatial Contact Force5/LConn1 -- Spatial Contact Force6/LConn1 -- Spatial Contact Force7/LConn1 -- Spatial Contact Force9/LConn1 -- Spatial Contact Force8/LConn1
  Spatial Contact Force7/RConn1 -- R7/LConn1
  Spatial Contact Force1/RConn1 -- R1/LConn1
  R9/RConn1 -- Revolute Joint9/RConn1
  Spatial Contact Force4/RConn1 -- R4/LConn1
  R8/RConn1 -- Revolute Joint8/RConn1
  Spatial Contact Force6/RConn1 -- R6/LConn1
  Spatial Contact Force2/RConn1 -- R2/LConn1
  Buje/RConn2 -- Revolute Joint3/LConn1
  Spatial Contact Force9/RConn1 -- R9/LConn1
  Buje/RConn4 -- Revolute Joint7/LConn1
  R6/RConn1 -- Revolute Joint6/RConn1
  Buje/LConn1 -- Revolute Joint1/LConn1
  R2/RConn1 -- Revolute Joint2/RConn1
  R5/RConn1 -- Revolute Joint5/RConn1
  Spatial Contact Force5/RConn1 -- R5/LConn1
  Buje/RConn3 -- Revolute Joint5/LConn1
  Spatial Contact Force8/RConn1 -- R8/LConn1
  Buje/LConn2 -- Revolute Joint2/LConn1
  Buje/LConn5 -- Revolute Joint8/LConn1
  Buje/RConn5 -- Revolute Joint9/LConn1
  _/RConn1 -- Rigid Transform/LConn1
  R4/RConn1 -- Revolute Joint4/RConn1
  Buje/LConn3 -- Revolute Joint4/LConn1
  R1/RConn1 -- Revolute Joint1/RConn1
  Buje/RConn1 -- Rigid Transform/RConn1
  R7/RConn1 -- Revolute Joint7/RConn1
  R3/RConn1 -- Revolute Joint3/RConn1
  Buje/LConn4 -- Revolute Joint6/LConn1
  Spatial Contact Force3/RConn1 -- R3/LConn1

== system Modelo_R2023b/Nexus/Nexus Robot/Wheel ω2 Front Right/DC_Motor Pololu 37DX70L 70:1 - 64 CPR ==
  U : Inport
  Angle Conversion : aerolibconvert2/Angle Conversion  IU=deg  OU=rad
  Electrical : Subsystem  mask{nomV=12}
      mask prompts: nomV "Nominal Voltage (V)"
  Mechanics : Subsystem
  PS-Simulink Converter : nesl_utility/PS-Simulink Converter  PhysicalDomain=network_engine_domain  SubClassName=ps_output  LeftPortType=input  RightPortType=output  PseudoPeriodic=off  Frequencies=[]  VectorFormat=1-D array  Unit=deg  AffineConversion=off
  PS-Simulink Converter1 : nesl_utility/PS-Simulink Converter  PhysicalDomain=network_engine_domain  SubClassName=ps_output  LeftPortType=input  RightPortType=output  PseudoPeriodic=off  Frequencies=[]  VectorFormat=1-D array  Unit=rad/s  AffineConversion=off
  PS-Simulink Converter2 : nesl_utility/PS-Simulink Converter  PhysicalDomain=network_engine_domain  SubClassName=ps_output  LeftPortType=input  RightPortType=output  PseudoPeriodic=off  Frequencies=[]  VectorFormat=1-D array  Unit=N*m  AffineConversion=off
  PS-Simulink Converter3 : nesl_utility/PS-Simulink Converter  PhysicalDomain=network_engine_domain  SubClassName=ps_output  LeftPortType=input  RightPortType=output  PseudoPeriodic=off  Frequencies=[]  VectorFormat=1-D array  Unit=A  AffineConversion=off
  Terminator : Terminator
  Terminator1 : Terminator
  Terminator2 : Terminator
  FW : PMIOPort  Side=Left
  Wheel : PMIOPort  Port=2  Side=Right
  θ : Outport
  wires:
  PS-Simulink Converter/1 -> Angle Conversion/1
  Angle Conversion/1 -> θ/1
  U/1 -> Electrical/1(U)
  PS-Simulink Converter1/1 -> Terminator/1
  PS-Simulink Converter2/1 -> Terminator1/1
  PS-Simulink Converter3/1 -> Terminator2/1
  connections:
  PS-Simulink Converter3/LConn1 -- Electrical/RConn2
  PS-Simulink Converter/LConn1 -- Mechanics/RConn2
  PS-Simulink Converter1/LConn1 -- Mechanics/RConn3
  Electrical/RConn1 -- PS-Simulink Converter2/LConn1 -- Mechanics/LConn2
  Mechanics/LConn1 -- FW/RConn1
  Wheel/RConn1 -- Mechanics/RConn1

== system Modelo_R2023b/Nexus/Nexus Robot/Wheel ω2 Front Right/Encoder ==
  In : Inport
  Difference : simulink/Discrete/Difference  ICPrevInput=0.0  OutMin=[]  OutMax=[]  OutDataType=fixdt(1, 16)  OutScaling=2^-10  DoSatur=off
  Gain : Gain  Gain=CPR/(2*pi)
  Gain1 : Gain  Gain=(2*pi)/CPR
  Gain2 : Gain  Gain=1/T_encoder
  Round : Rounding  Operator=fix
  Out : Outport
  wires:
  Round/1 -> Gain1/1
  Gain/1 -> Round/1
  Gain1/1 -> Difference/1
  In/1 -> Gain/1
  Difference/1 -> Gain2/1
  Gain2/1 -> Out/1

== system Modelo_R2023b/Nexus/Nexus Robot/Wheel ω2 Front Right/PID Controller ==
  ω_ref : Inport
  ω : Inport  Port=2
  Discrete Derivative : simulink/Discrete/Discrete Derivative  gainval=1.0  ICPrevScaledInput=0.0  OutMin=[]  OutMax=[]  OutDataType=fixdt(1, 16)  OutScaling=2^-10  DoSatur=off
  Discrete-Time Integrator1 : DiscreteIntegrator  SampleTime=MOTOR_Period_T  ICPrevOutput=DiscIntNeverNeededParam  ICPrevScaledInput=DiscIntNeverNeededParam
  Gain : Gain  Gain=4096/12
  Gain1 : Gain  Gain=DC_Motor_P
  Gain2 : Gain  Gain=DC_Motor_I
  Gain3 : Gain  Gain=DC_Motor_D
  Sum : Sum  Inputs=+-|
  Sum1 : Sum  Inputs=+++
  ω_u : Outport
  wires:
  Gain/1 -> ω_u/1
  ω/1 -> Sum/2
  Gain2/1 -> Discrete-Time Integrator1/1
  Sum/1 -> Gain3/1, Gain1/1, Gain2/1  "error"
  Sum1/1 -> Gain/1  "ω_v"
  ω_ref/1 -> Sum/1
  Discrete-Time Integrator1/1 -> Sum1/2
  Gain1/1 -> Sum1/1
  Discrete Derivative/1 -> Sum1/3
  Gain3/1 -> Discrete Derivative/1
